simulink model "sixthone"  (R2020b)
settings: Solver=VariableStepAuto  StartTime=0.0  StopTime=10.0  MaxStep=0.001  RelTol=1e-3
model workspace: external: MATLAB File C:\Users\deves\MATLAB\Projects\problem6\data6.m (data not in the file)
settings Model: Creator=deves  LastModifiedBy=deves

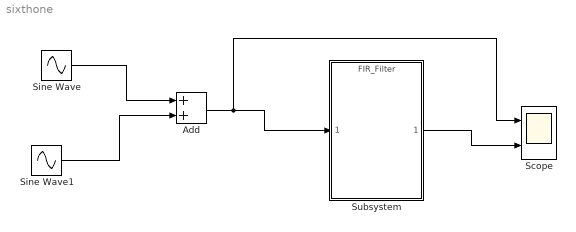
== system sixthone ==
  Add : Sum
  Scope : Scope  NumInputPorts=2
  Sine Wave : Sin  SampleTime=0
  Sine Wave1 : Sin  Frequency=500  SampleTime=0
  Subsystem : ModelReference  ModelNameDialog=FIR_Filter  SimulationMode=Normal  ModelReferenceVersion=1.1
  wires:
  Add/1 -> Scope/1, Subsystem/1
  Subsystem/1 -> Scope/2
  Sine Wave1/1 -> Add/2
  Sine Wave/1 -> Add/1
